simulink model "adaptiv_puls_elimination"  (Simulink 7.1)
settings: Solver=ode45  StartTime=0.0  StopTime=2000  RelTol=1e-3
values from neighbouring files (symbols this model uses):
  n_koeff = 32    [EHK_adaptivePuls_online_simulation.m]    (also in EHK_adaptpulsonline.m)
  TS = Ts    (= 0.1)    [EHK_adaptivePuls_online_simulation.m]    (also in EHK_adaptpulsonline.m = 0.333333333333)
libraries: dspadpt3 x1
settings Model: Creator=svenhoffmann  LastModifiedBy=bauernfeind  ExtModeAutoUpdateStatusClock=off
settings DataIOCC: SignalLoggingName=sigsOut
settings DebuggingCC: SaveWithParameterizedLinksMsg=none  SignalResolutionControl=TryResolveAllWithWarning  SolverPrmCheckMsg=none  MultiTaskDSMMsg=warning  MultiTaskCondExecSysMsg=none  StrictBusMsg=None
settings HardwareCC: TargetUnknown=on
settings RTWCC: IncludeERTFirstTime=on
settings GRTTargetCC: TargetFcnLib=ansi_tfl_tmw.mat

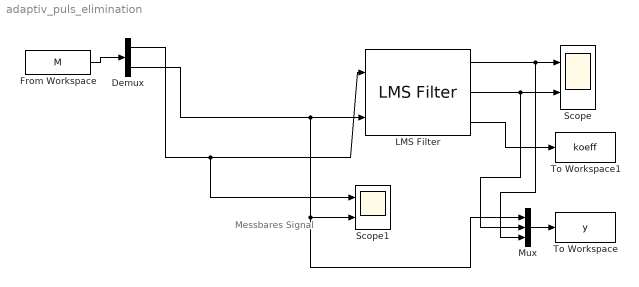
== system adaptiv_puls_elimination ==
  note: Messbares
      | Signal
  Demux : Demux  Outputs=2
  From Workspace : FromWorkspace  VariableName=M  SampleTime=TS  OutputAfterFinalValue=Setting to zero
  LMS Filter : dspadpt3/LMS Filter  DialogController=dspDDGCreate  DialogControllerArgs=DataTag0  Algo=Normalized LMS  L=n_koeff  stepflag=Dialog  mu=mu  leakage=1.0  ic=0  Adapt=off  resetflag=None  weights=on  secondCoeffMode=User-defined  secondCoeffWordLength=2  secondCoeffFracLength=15  accum2Mode=User-defined  accum2FracLength=20  prodOutput2Mode=User-defined  prodOutput2FracLength=20  prodOutput3Mode=User-defined  prodOutput3FracLength=20  prodOutput4Mode=User-defined  prodOutput4FracLength=20  quotientMode=User-defined  quotientFracLength=20  roundingMode=Floor  overflowMode=off  addnparflag=off
  Mux : Mux  Inputs=3
  Scope : Scope  NumInputPorts=2
      settings: YMin=-7.5~-10  YMax=7.5~10  SaveName=ScopeData2
  Scope1 : Scope  NumInputPorts=2
      settings: YMin=-5~-30  YMax=7.5~30
  To Workspace : ToWorkspace  VariableName=y  SampleTime=-1  SaveFormat=Array
  To Workspace1 : ToWorkspace  VariableName=koeff  SampleTime=-1  SaveFormat=Array
      settings: MaxDataPoints=1
  wires:
  LMS Filter/1 -> Scope/1, Mux/3
  LMS Filter/2 -> Scope/2, Mux/2
  LMS Filter/3 -> To Workspace1/1
  Mux/1 -> To Workspace/1
  From Workspace/1 -> Demux/1
  Demux/2 -> LMS Filter/2, Scope1/2, Mux/1
  Demux/1 -> LMS Filter/1, Scope1/1
